simulink model "ELEC3114_Lab2_QuanserDCMotorSRV02_Template_2026"  (R2025b)
settings: Solver=ode1  StartTime=0.0  StopTime=Inf  FixedStep=0.002  RelTol=1e-3
values from neighbouring files (symbols this model uses):
  fc = 10    [ELEC3114_Lab2_New.m]
  zeta = 0.707    [ELEC3114_Lab2_New.m]
undefined symbols (not defined in the file or in its folder): National_Instruments, PCIe
libraries: sldrtlib x3, simulink x1
settings Model: SimulationMode=external  ExtModeTrigDuration=5000  Creator=MyProject  LastModifiedBy=My Project
settings SolverCC: AlgebraicLoopSolver=TrustRegion
settings DataIOCC: SaveOutput=off  SignalLogging=off  DSMLogging=off  SaveTime=off  ReturnWorkspaceOutputs=off
settings DebuggingCC: UnconnectedInputMsg=warning  UnconnectedOutputMsg=warning  UnconnectedLineMsg=warning
settings HardwareCC: ProdBitPerLong=64.0  ProdHWDeviceType=Intel->x86-64 (Linux 64)
settings ModelReferenceCC: EnableRefExpFcnMdlSchedulingChecks=on
settings RTWCC: SystemTargetFile=sldrt.tlc  TemplateMakefile=sldrt.tmf  RTWCompilerOptimization=on  GPUComputeCapability=3.5  Description=Simulink Desktop Real-Time
settings CodeAppCC: MaxIdLength=95.0
settings SimulinkDesktopRealTimeCC: ExtModeTransport=0.0  ExtModeStaticAllocSize=1000000.0  TargetLibSuffix=_sldrt.a  TargetPreCompLibLocation=C:\Program Files\MATLAB\R2025b\toolbox\sldrt\lib\win64  MultiwordLength=2048.0  DynamicStringBufferSize=256.0  ParMdlRefBuildCompliant=on  PreserveMATLABNamespacesInGeneratedCode=on  SubcomponentCodeInterfacePackaging=Reusable function

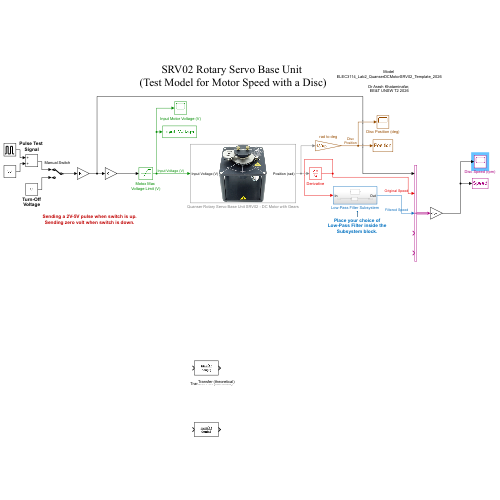
[thumbnail: Simulink's stored preview of the top-level diagram]
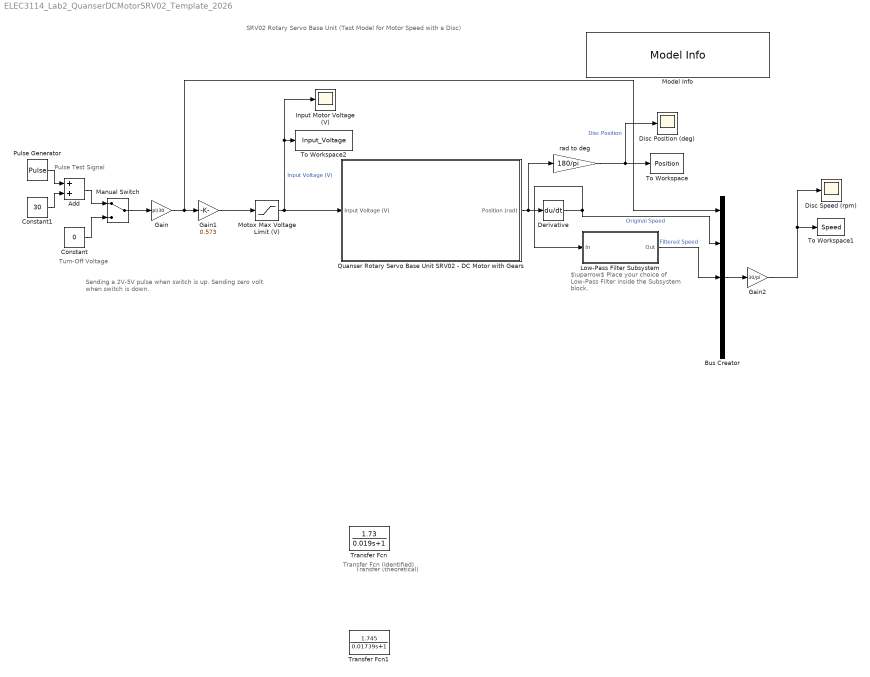
== system ELEC3114_Lab2_QuanserDCMotorSRV02_Template_2026 ==
  note: Transfer (theoretical)
  note: Transfer Fcn (Identified)
  note: SRV02 Rotary Servo Base Unit
      | (Test Model for Motor Speed with a Disc)
  note: Sending a 2V-5V pulse when switch is up.
      | Sending zero volt when switch is down.
  note: Pulse Test
      | Signal
  note: Turn-Off
      | Voltage
  note: $\uparrow$
      | Place your choice of
      | Low-Pass Filter inside the Subsystem block.
  Add : Sum
  Bus Creator : BusCreator  Inputs=5
  Constant : Constant  Value=0
  Constant1 : Constant  Value=30
  Derivative : Derivative
  Disc Position (deg) : Scope
      settings: ActiveDisplayYMinimum=708.55112441031577  ActiveDisplayYMaximum=725.37633701535185  YLabel=Position (deg)  DataLoggingVariableName=ScopeData3  DataLoggingSaveFormat=Array
  Disc Speed (rpm) : Scope
      settings: Title=Disc Speed/Velocity  ActiveDisplayYMinimum=-7.4999999999999982  ActiveDisplayYMaximum=67.5  YLabel=Speed (rad/s)
  Gain : Gain  Gain=pi/30
  Gain1 : Gain  Gain=0.573
  Gain2 : Gain  Gain=30/pi
  Input Motor Voltage (V) : Scope
      settings: Title=Input Motor Voltage  ActiveDisplayYMinimum=0  ActiveDisplayYMaximum=6  YLabel=Voltage (V)  DataLoggingVariableName=ScopeData4
  Low-Pass Filter Subsystem : Subsystem
  Manual Switch : ManualSwitch
  Model Info : simulink/Model-Wide Utilities/Model Info  Frame=off  DisplayStringWithTags=|  HorizontalTextAlignment=Center  LeftAlignmentValue=0.5
      | Model 
      | %<ModelName>
      | 
      | Dr Arash Khataminafar, 
      | EE&T UNSW T2 2026
  Motox Max Voltage Limit (V) : Saturate  UpperLimit=8  LowerLimit=-8
  Pulse Generator : DiscretePulseGenerator  PulseType=Time based  Amplitude=30  PulseWidth=50  PhaseDelay=1
  Quanser Rotary Servo Base Unit SRV02 - DC Motor with Gears : Subsystem
      mask Display: image('Quanser Rotary Base Unit SRV02.png', [0,0,0,0,60,100]);
  To Workspace : ToWorkspace  VariableName=Position  SaveFormat=Structure With Time  SampleTime=0.002
  To Workspace1 : ToWorkspace  VariableName=Speed  SaveFormat=Structure With Time  SampleTime=0.002
  To Workspace2 : ToWorkspace  VariableName=Input_Voltage  SaveFormat=Structure With Time  SampleTime=0.002
  Transfer Fcn : TransferFcn  Numerator=[1.73]  Denominator=[0.019 1]
  Transfer Fcn1 : TransferFcn  Numerator=[1.745]  Denominator=[0.01739 1]
  rad to deg : Gain  Gain=180/pi
  wires:
  rad to deg/1 -> To Workspace/1, Disc Position (deg)/1  "Disc Position"
  Constant/1 -> Manual Switch/2
  Manual Switch/1 -> Gain/1
  Low-Pass Filter Subsystem/1(Out) -> Bus Creator/3  "Filtered Speed"
  Derivative/1 -> Low-Pass Filter Subsystem/1(In), Bus Creator/2  "Original Speed"
  Bus Creator/1 -> Gain2/1
  Pulse Generator/1 -> Add/1
  Constant1/1 -> Add/2
  Add/1 -> Manual Switch/1
  Motox Max Voltage Limit (V)/1 -> Quanser Rotary Servo Base Unit SRV02 - DC Motor with Gears/1(Input Voltage (V)), Input Motor Voltage (V)/1, To Workspace2/1  "Input Voltage (V)"
  Quanser Rotary Servo Base Unit SRV02 - DC Motor with Gears/1(Position (rad)) -> rad to deg/1, Derivative/1
  Gain/1 -> Bus Creator/1, Gain1/1
  Gain1/1 -> Motox Max Voltage Limit (V)/1
  Gain2/1 -> Disc Speed (rpm)/1, To Workspace1/1

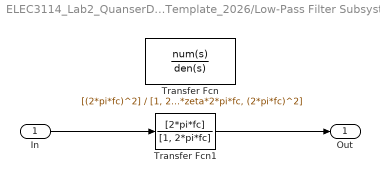
== system ELEC3114_Lab2_QuanserDCMotorSRV02_Template_2026/Low-Pass Filter Subsystem ==
  In : Inport
  Transfer Fcn : TransferFcn  Numerator=[(2*pi*fc)^2]  Denominator=[1, 2*zeta*2*pi*fc, (2*pi*fc)^2]
  Transfer Fcn1 : TransferFcn  Numerator=[2*pi*fc]  Denominator=[1, 2*pi*fc]
  Out : Outport
  wires:
  In/1 -> Transfer Fcn1/1
  Transfer Fcn1/1 -> Out/1

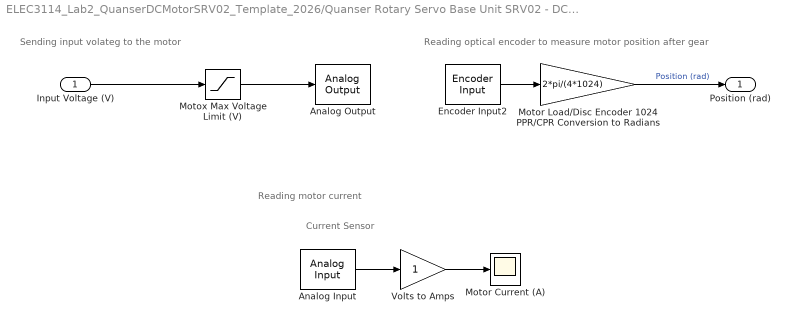
== system ELEC3114_Lab2_QuanserDCMotorSRV02_Template_2026/Quanser Rotary Servo Base Unit SRV02 - DC Motor with Gears ==
  note: Reading motor current
  note: Reading optical encoder to measure motor position after gear
  note: Sending input volateg to the motor
  note: Current
      | Sensor
  Input Voltage (V) : Inport
  Analog Input : sldrtlib/Analog Input  SampleTime=0.002  MaxMissedTicks=10  ShowMissedTicks=off  YieldWhenWaiting=off  DrvName=National_Instruments/PCIe-6351  DrvAddress=4294967295  DrvOptions=[1 0 0 2 2 2 2]  Channels=1  RangeMode=1  VoltRange=1  DataType=1
      settings: AttributesFormatString=National Instruments\nPCIe-6351 [auto]
  Analog Output : sldrtlib/Analog Output  SampleTime=0.002  MaxMissedTicks=10  ShowMissedTicks=off  YieldWhenWaiting=off  DrvName=National_Instruments/PCIe-6351  DrvAddress=4294967295  DrvOptions=[1 0 0 2 2 2 2]  Channels=1  RangeMode=1  VoltRange=1  InitialValue=0  FinalValue=0
      settings: AttributesFormatString=National Instruments\nPCIe-6351 [auto]
  Encoder Input2 : sldrtlib/Encoder Input  SampleTime=0.002  MaxMissedTicks=10  ShowMissedTicks=off  YieldWhenWaiting=off  DrvName=National_Instruments/PCIe-6351  DrvAddress=4294967295  DrvOptions=[1 0 0 2 2 2 2]  Channels=[1]  QuadMode=3  IndexPulse=2  InputFilter=Inf  DataType=1
      settings: AttributesFormatString=National Instruments\nPCIe-6351 [auto]
  Motor Current (A) : Scope
      settings: ActiveDisplayYMinimum=-1.9062414914262209  ActiveDisplayYMaximum=2.7285271128026514
  Motor Load/Disc Encoder 1024 PPR/CPR Conversion to Radians : Gain  Gain=2*pi/(4*1024)  SaturateOnIntegerOverflow=on  OutDataTypeStr=Inherit: Same as input  ParamDataTypeStr=Inherit: Same as input
  Motox Max Voltage Limit (V) : Saturate  UpperLimit=8  LowerLimit=-8
  Volts to Amps : Gain  OutDataTypeStr=Inherit: Same as input  ParamDataTypeStr=Inherit: Same as input
  Position (rad) : Outport
  wires:
  Encoder Input2/1 -> Motor Load/Disc Encoder 1024 PPR/CPR Conversion to Radians/1
  Motor Load/Disc Encoder 1024 PPR/CPR Conversion to Radians/1 -> Position (rad)/1  "Position (rad)"
  Volts to Amps/1 -> Motor Current (A)/1
  Analog Input/1 -> Volts to Amps/1
  Input Voltage (V)/1 -> Motox Max Voltage Limit (V)/1
  Motox Max Voltage Limit (V)/1 -> Analog Output/1
